simulink model "Ecuacion_Diferencial_Codigo_Ejercicio_5"  (R2017b)
settings: Solver=ode1  StartTime=0.0  StopTime=10.0  RelTol=1e-3
settings Model: Creator=Elmer  LastModifiedBy=Elmer

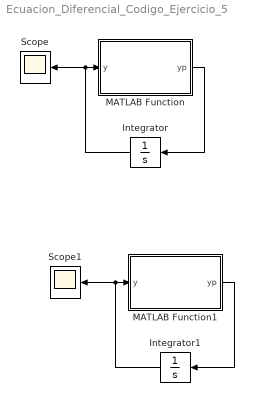
== system Ecuacion_Diferencial_Codigo_Ejercicio_5 ==
  Integrator : Integrator  InitialCondition=1
  Integrator1 : Integrator  InitialCondition=0.5
  MATLAB Function : MATLAB Function  TreatAsAtomicUnit=on
  MATLAB Function1 : MATLAB Function  TreatAsAtomicUnit=on
  Scope : Scope
  Scope1 : Scope
  wires:
  MATLAB Function/1(yp) -> Integrator/1
  Integrator/1 -> Scope/1, MATLAB Function/1(y)
  Integrator1/1 -> Scope1/1, MATLAB Function1/1(y)
  MATLAB Function1/1(yp) -> Integrator1/1

== matlab function Ecuacion_Diferencial_Codigo_Ejercicio_5/MATLAB Function1 ==
  data: y input; yp output
function yp = fcn(y)
yp= (y-1)^2;

== matlab function Ecuacion_Diferencial_Codigo_Ejercicio_5/MATLAB Function ==
  data: y input; yp output
function yp = fcn(y)
yp= y^2 - 4;
